simulink model "untitled"  (R2024b)
settings: Solver=VariableStepAuto  StartTime=0.0  StopTime=10.0  RelTol=1e-3
undefined symbols (not defined in the file or in its folder): DiscIntNeverNeededParam
libraries: robotmobilelib x1
settings Model: Creator=johan  LastModifiedBy=johan

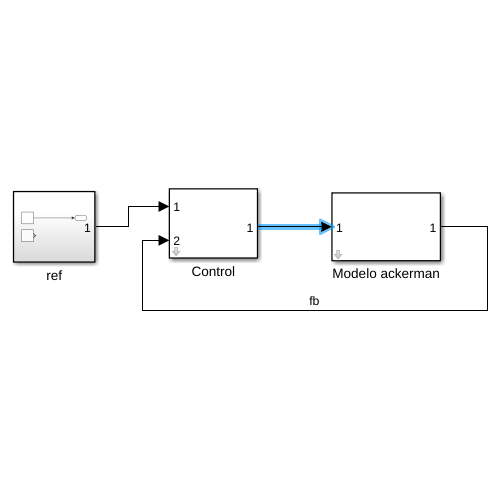
[thumbnail: Simulink's stored preview of the top-level diagram]
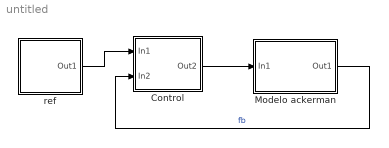
== system untitled ==
  Control : Subsystem  mask{Kp=15, Ki=0}
      mask prompts: Kp "Proportional (Kp):"; Ki "Integral (Ki):"
  Modelo ackerman : Subsystem  mask{wheel_base=1, speed_limit=10, angular_limit=pi/4}
      mask prompts: wheel_base "Diametro rueda:"; speed_limit "Limite velocidad:"; angular_limit "Limite angular:"
  ref : Subsystem
  wires:
  Control/1(Out2) -> Modelo ackerman/1(In1)
  Modelo ackerman/1(Out1) -> Control/2(In2)  "fb"
  ref/1(Out1) -> Control/1(In1)

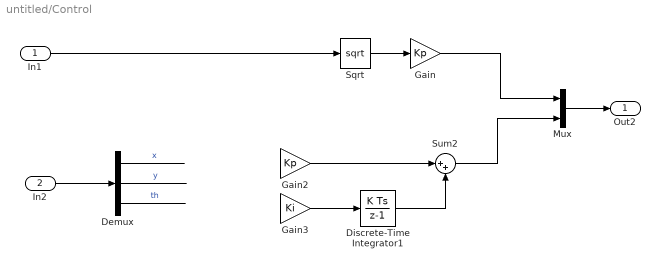
== system untitled/Control ==
  In1 : Inport
  In2 : Inport  Port=2
  Demux : Demux  Outputs=3
  Discrete-Time Integrator1 : DiscreteIntegrator  SampleTime=-1  ICPrevOutput=DiscIntNeverNeededParam  ICPrevScaledInput=DiscIntNeverNeededParam
  Gain : Gain  Gain=Kp
  Gain2 : Gain  Gain=Kp
  Gain3 : Gain  Gain=Ki
  Mux : Mux  Inputs=2
  Sqrt : Sqrt
  Sum2 : Sum  Inputs=|++
  Out2 : Outport
  wires:
  Gain/1 -> Mux/1
  In1/1 -> Sqrt/1
  In2/1 -> Demux/1
  Demux/1 -> ?  "x"
  Demux/2 -> ?  "y"
  Demux/3 -> ?  "th"
  Mux/1 -> Out2/1
  ? -> Gain3/1
  ? -> Gain2/1
  Gain2/1 -> Sum2/1
  Gain3/1 -> Discrete-Time Integrator1/1
  Discrete-Time Integrator1/1 -> Sum2/2
  Sum2/1 -> Mux/2
  Sqrt/1 -> Gain/1

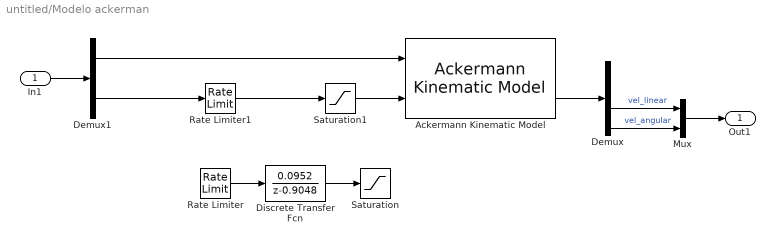
== system untitled/Modelo ackerman ==
  In1 : Inport
  Ackermann Kinematic Model : robotmobilelib/Ackermann Kinematic Model  WheelBase=wheel_base  VehicleSpeedRange=[-speed_limit speed_limit]  MaxSteeringAngle=angular_limit  InitialState=[0; 0; 0; 0]  SimulateUsing=Interpreted execution
  Demux : Demux
  Demux1 : Demux  Outputs=2
  Discrete Transfer Fcn : DiscreteTransferFcn  Numerator="[0    0.0952]"  Denominator="[1.0000   -0.9048]"
  Mux : Mux  Inputs=2
  Rate Limiter : RateLimiter  RisingSlewLimit=0.6  FallingSlewLimit=-0.6  SampleTimeMode=inherited
  Rate Limiter1 : RateLimiter  RisingSlewLimit=0.6  FallingSlewLimit=-0.6  SampleTimeMode=inherited
  Saturation : Saturate
  Saturation1 : Saturate
  Out1 : Outport
  wires:
  Demux1/1 -> Ackermann Kinematic Model/1
  Ackermann Kinematic Model/2 -> Demux/1
  Demux1/2 -> Rate Limiter1/1
  Demux/3 -> Mux/1  "vel_linear"
  Demux/4 -> Mux/2  "vel_angular"
  ? -> Rate Limiter/1
  Discrete Transfer Fcn/1 -> Saturation/1
  Rate Limiter/1 -> Discrete Transfer Fcn/1
  Rate Limiter1/1 -> Saturation1/1
  Saturation1/1 -> Ackermann Kinematic Model/2
  In1/1 -> Demux1/1
  Mux/1 -> Out1/1

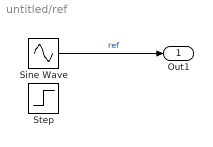
== system untitled/ref ==
  Sine Wave : Sin  SampleTime=0
  Step : Step  After=pi/8  SampleTime=0
  Out1 : Outport
  wires:
  Sine Wave/1 -> Out1/1  "ref"
